simulink model "ThreePhaseVectorControl"  (R2020a)
settings: Solver=ode15s  StartTime=0.0  StopTime=2.5  MaxStep=1e-6  RelTol=1e-6
model workspace (MAT data in the model file):
  frequency = 1
values from neighbouring files (symbols this model uses):
  Buffer = 500    [PLLFYP.m]
  Ki_PLL = 0.005    [PLLFYP.m]
  Kp_PLL = 0.05    [PLLFYP.m]
  Kp_VSC = 500    [PLLFYP.m]
  Lf = 0.005    [PLLFYP.m]
  Lg = XR*Rg/(100*pi)    [PLLFYP.m]
  MPM_Ts = 1/5000    (= 0.0002)    [PLLFYP.m]
  Rf = 0.1    [PLLFYP.m]
  Rg = sqrt((1/(1+XR^2))*((500^2)/(Pn*SCR))^2)    [PLLFYP.m]
  Vdc = 2000    [PLLFYP.m]
  wL = 2*pi*50*Lf    (= 1.57079632679)    [PLLFYP.m]
  wn = 3000    [PLLFYP.m]
  zeta = 0.707    [PLLFYP.m]
undefined symbols (not defined in the file or in its folder): Ki_PQ, Kp_PQ, mpm_wc, plecs, Q, Q_KF, R, wb, wc, wc1, wc2
libraries: powerlib_meascontrol x57, powerlib x25, simulink x4, eeStairGenerator x4, powerlib_extras x2, cstblocks x2
(part 2 of 4)

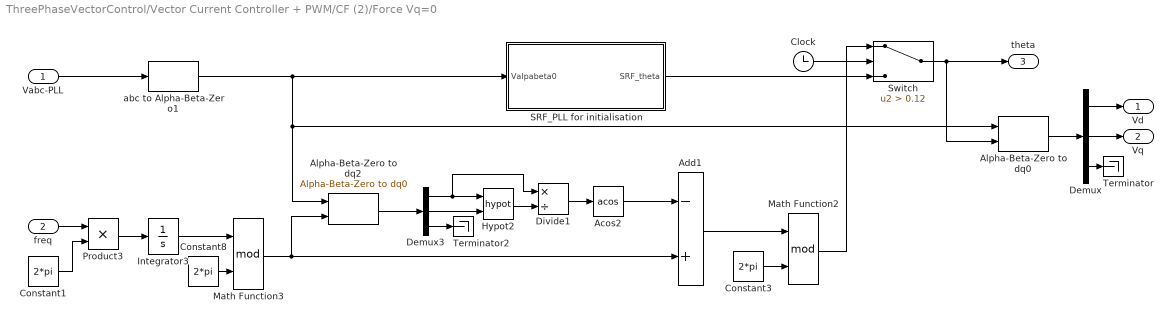
== system ThreePhaseVectorControl/Vector Current Controller + PWM/CF (2)/Force Vq=0 ==
  Vabc-PLL : Inport
  freq : Inport  Port=2
  Acos2 : Trigonometry  Operator=acos
  Add1 : Sum  Inputs=-+
  Alpha-Beta-Zero to dq0 : powerlib_meascontrol/Transformations/Alpha-Beta-Zero to dq0  Alignment=Aligned with phase A axis
  Alpha-Beta-Zero to dq2 : powerlib_meascontrol/Transformations/Alpha-Beta-Zero to dq0  Alignment=Aligned with phase A axis
  Clock : Clock
  Constant1 : Constant  Value=2*pi
  Constant3 : Constant  Value=2*pi
  Constant8 : Constant  Value=2*pi
  Demux : Demux  Outputs=3
  Demux3 : Demux  Outputs=3
  Divide1 : Product  Inputs=*/
  Hypot2 : Math  Operator=hypot  SaturateOnIntegerOverflow=on
  Integrator3 : Integrator  UpperSaturationLimit=2*pi  LowerSaturationLimit=0  IgnoreLimit=on
  Math Function2 : Math  Operator=mod  SignedPower=on  SaturateOnIntegerOverflow=on
  Math Function3 : Math  Operator=mod  SignedPower=on  SaturateOnIntegerOverflow=on
  Product3 : Product  RndMeth=Zero
  SRF_PLL for initialisation : Subsystem
  Switch : Switch  Criteria=u2 > Threshold  Threshold=0.12
  Terminator : Terminator
  Terminator2 : Terminator
  abc to Alpha-Beta-Zero1 : powerlib_meascontrol/Transformations/abc to Alpha-Beta-Zero
  Vd : Outport
  Vq : Outport  Port=2
  theta : Outport  Port=3  VectorParamsAs1DForOutWhenUnconnected=off
  wires:
  Add1/1 -> Math Function2/1
  Alpha-Beta-Zero to dq2/1 -> Demux3/1
  Demux3/3 -> Terminator2/1
  Constant3/1 -> Math Function2/2
  Math Function2/1 -> Switch/1
  Clock/1 -> Switch/2
  SRF_PLL for initialisation/1(SRF_theta) -> Switch/3
  Switch/1 -> theta/1, Alpha-Beta-Zero to dq0/2
  Divide1/1 -> Acos2/1
  Hypot2/1 -> Divide1/2
  Acos2/1 -> Add1/1
  Demux3/1 -> Hypot2/1, Divide1/1
  Demux3/2 -> Hypot2/2
  Vabc-PLL/1 -> abc to Alpha-Beta-Zero1/1
  Integrator3/1 -> Math Function3/1
  Constant1/1 -> Product3/2
  Product3/1 -> Integrator3/1
  Constant8/1 -> Math Function3/2
  freq/1 -> Product3/1
  Math Function3/1 -> Alpha-Beta-Zero to dq2/2, Add1/2
  abc to Alpha-Beta-Zero1/1 -> SRF_PLL for initialisation/1(Valpabeta0), Alpha-Beta-Zero to dq0/1, Alpha-Beta-Zero to dq2/1
  Alpha-Beta-Zero to dq0/1 -> Demux/1
  Demux/3 -> Terminator/1
  Demux/2 -> Vq/1
  Demux/1 -> Vd/1

== system ThreePhaseVectorControl/Vector Current Controller + PWM/CF (2)/MPM ==
  va : Inport
  Buffer : Buffer  N=Buffer  V=Overlap  ic=zeros(Buffer,1)  OutputFrames=off
  Clock3 : Clock
      settings: Decimation=100
  Constant : Constant  Value=Buffer/2
  Constant1 : Constant  Value=50
  Constant2 : Constant  Value=MPM_Ts
  Constant4 : Constant  Value=50
  MPM method : MATLAB Function  TreatAsAtomicUnit=on
  Scope2 : Scope
  Switch3 : Switch  Criteria=u2 > Threshold  Threshold=0.1
  Zero-Order Hold : ZeroOrderHold  SampleTime=MPM_Ts
  MPM freq : Outport
  wires:
  Constant/1 -> MPM method/2(L)
  Zero-Order Hold/1 -> Scope2/1, Buffer/1
  Constant1/1 -> MPM method/4(freq_guess)
  Buffer/1 -> MPM method/1(x)
  Clock3/1 -> Switch3/2
  Constant4/1 -> Switch3/3
  Constant2/1 -> MPM method/3(timestep)
  MPM method/1(outputfreq) -> Switch3/1
  va/1 -> Zero-Order Hold/1
  Switch3/1 -> MPM freq/1

== system ThreePhaseVectorControl/Vector Current Controller + PWM/CF (2)/SRF PLL ==
  Vabc : Inport
  1/(2*pi) : Step  Time=0  After=1/(2*pi)  SampleTime=0
  Add : Sum  Inputs=+-
  Add1 : Sum
  Constant : Constant  Value=2*pi
  Demux : Demux  Outputs=3
  Gain : Gain  Gain=Kp_PLL
  Integrator : Integrator  UpperSaturationLimit=2*pi  LowerSaturationLimit=0  IgnoreLimit=on
  Math Function : Math  Operator=mod  SignedPower=on  SaturateOnIntegerOverflow=on
  PI Controller : TransferFcn  Numerator=[1 Ki_PLL]  Denominator=[1 0]
  Product : Product  RndMeth=Zero
  Terminator : Terminator
  Terminator1 : Terminator
  abc to dq0 : powerlib_meascontrol/Transformations/abc to dq0  Alignment=Aligned with phase A axis
  q reference : Step  Time=0  After=0  SampleTime=0
  w0 : Step  Time=0  After=2*pi*50  SampleTime=0
  frequency : Outport
  delta_w0 : Outport  Port=2
  wires:
  Vabc/1 -> abc to dq0/1
  Integrator/1 -> Math Function/1
  Gain/1 -> PI Controller/1
  Add1/1 -> Product/2, Integrator/1
  Demux/2 -> Add/1
  w0/1 -> Add1/2
  q reference/1 -> Add/2
  1/(2*pi)/1 -> Product/1
  Product/1 -> frequency/1
  PI Controller/1 -> Add1/1, delta_w0/1
  Constant/1 -> Math Function/2
  Demux/3 -> Terminator/1
  Add/1 -> Gain/1
  abc to dq0/1 -> Demux/1
  Math Function/1 -> abc to dq0/2
  Demux/1 -> Terminator1/1

== system ThreePhaseVectorControl/Vector Current Controller + PWM/CF 2/MPM ==
  va : Inport
  Buffer : Buffer  N=500  V=499  ic=zeros(500,1)  OutputFrames=off
  Clock3 : Clock
      settings: Decimation=100
  Constant : Constant  Value=250
  Constant1 : Constant  Value=50
  Constant2 : Constant  Value=MPM_Ts
  Constant4 : Constant  Value=50
  MPM method : MATLAB Function  TreatAsAtomicUnit=on
  Scope2 : Scope
  Switch3 : Switch  Criteria=u2 > Threshold  Threshold=0.12
  Zero-Order Hold : ZeroOrderHold  SampleTime=MPM_Ts
  MPM freq : Outport
  wires:
  Constant/1 -> MPM method/2(L)
  Zero-Order Hold/1 -> Scope2/1, Buffer/1
  Constant1/1 -> MPM method/4(freq_guess)
  Buffer/1 -> MPM method/1(x)
  Clock3/1 -> Switch3/2
  Constant4/1 -> Switch3/3
  Constant2/1 -> MPM method/3(timestep)
  MPM method/1(outputfreq) -> Switch3/1
  va/1 -> Zero-Order Hold/1
  Switch3/1 -> MPM freq/1

== system ThreePhaseVectorControl/Vector Current Controller + PWM/CF 2/MPM (forcing Vq=0) ==
  Vabc-PLL : Inport
  MPM theta : Inport  Port=2
  Acos2 : Trigonometry  Operator=acos
  Add1 : Sum  Inputs=-+
  Alpha-Beta-Zero to dq2 : powerlib_meascontrol/Transformations/Alpha-Beta-Zero to dq0  Alignment=Aligned with phase A axis
  Clock : Clock
  Constant3 : Constant  Value=2*pi
  Demux3 : Demux  Outputs=3
  Divide1 : Product  Inputs=*/
  Hypot2 : Math  Operator=hypot  SaturateOnIntegerOverflow=on
  Math Function2 : Math  Operator=mod  SignedPower=on  SaturateOnIntegerOverflow=on
  SRF-PLL for initialization : Subsystem
  Switch : Switch  Criteria=u2 > Threshold  Threshold=0.12
  Terminator2 : Terminator
  abc to Alpha-Beta-Zero1 : powerlib_meascontrol/Transformations/abc to Alpha-Beta-Zero
  MPM_theta : Outport  VectorParamsAs1DForOutWhenUnconnected=off
  wires:
  Add1/1 -> Math Function2/1
  Alpha-Beta-Zero to dq2/1 -> Demux3/1
  Demux3/3 -> Terminator2/1
  Constant3/1 -> Math Function2/2
  Math Function2/1 -> Switch/1
  Clock/1 -> Switch/2
  SRF-PLL for initialization/1(SRF_theta) -> Switch/3
  abc to Alpha-Beta-Zero1/1 -> Alpha-Beta-Zero to dq2/1, SRF-PLL for initialization/1(VaB0)
  Switch/1 -> MPM_theta/1
  MPM theta/1 -> Alpha-Beta-Zero to dq2/2, Add1/2
  Divide1/1 -> Acos2/1
  Hypot2/1 -> Divide1/2
  Acos2/1 -> Add1/1
  Demux3/1 -> Hypot2/1, Divide1/1
  Demux3/2 -> Hypot2/2
  Vabc-PLL/1 -> abc to Alpha-Beta-Zero1/1

== system ThreePhaseVectorControl/Vector Current Controller + PWM/CF 2/SRF PLL ==
  abc : Inport
  wt : Inport  Port=2
  1/(2*pi) : Step  Time=0  After=1/(2*pi)  SampleTime=0
  Add : Sum  Inputs=+-
  Add1 : Sum
  Constant : Constant  Value=2*pi
  Demux : Demux  Outputs=3
  Gain : Gain  Gain=Kp_PLL
  Integrator : Integrator  UpperSaturationLimit=2*pi  LowerSaturationLimit=0  IgnoreLimit=on
  Math Function : Math  Operator=mod  SignedPower=on  SaturateOnIntegerOverflow=on
  PI Controller : TransferFcn  Numerator=[1 Ki_PLL]  Denominator=[1 0]
  Product : Product  RndMeth=Zero
  Terminator : Terminator
  abc to dq0 : powerlib_meascontrol/Transformations/abc to dq0  Alignment=Aligned with phase A axis
  q reference : Step  Time=0  After=0  SampleTime=0
  w0 : Step  Time=0  After=2*pi*50  SampleTime=0
  Vd : Outport  VectorParamsAs1DForOutWhenUnconnected=off
  Vq : Outport  Port=2  VectorParamsAs1DForOutWhenUnconnected=off
  delta_w0 : Outport  Port=3
  frequency : Outport  Port=4
  theta : Outport  Port=5
  wires:
  abc/1 -> abc to dq0/1
  Gain/1 -> PI Controller/1
  Add1/1 -> Integrator/1, Product/2
  Demux/2 -> Vq/1, Add/1
  w0/1 -> Add1/2
  Demux/1 -> Vd/1
  q reference/1 -> Add/2
  1/(2*pi)/1 -> Product/1
  Product/1 -> frequency/1
  PI Controller/1 -> Add1/1, delta_w0/1
  Demux/3 -> Terminator/1
  Add/1 -> Gain/1
  abc to dq0/1 -> Demux/1
  wt/1 -> abc to dq0/2
  Constant/1 -> Math Function/2
  Integrator/1 -> Math Function/1
  Math Function/1 -> theta/1

== system ThreePhaseVectorControl/Vector Current Controller + PWM/FFT_PLL/MPM (forcing Vq=0) ==
  Vabc-PLL : Inport
  FFT theta : Inport  Port=2
  Acos2 : Trigonometry  Operator=acos
  Add1 : Sum  Inputs=-+
  Alpha-Beta-Zero to dq2 : powerlib_meascontrol/Transformations/Alpha-Beta-Zero to dq0  Alignment=Aligned with phase A axis
  Alpha-Beta-Zero to dq3 : powerlib_meascontrol/Transformations/Alpha-Beta-Zero to dq0  Alignment=Aligned with phase A axis
  Clock : Clock
  Constant3 : Constant  Value=2*pi
  Demux3 : Demux  Outputs=3
  Demux4 : Demux  Outputs=3
  Divide1 : Product  Inputs=*/
  Hypot2 : Math  Operator=hypot  SaturateOnIntegerOverflow=on
  Math Function2 : Math  Operator=mod  SignedPower=on  SaturateOnIntegerOverflow=on
  SRF-PLL for initialization : Subsystem
  Switch : Switch  Criteria=u2 > Threshold  Threshold=0.12
  Terminator2 : Terminator
  Terminator3 : Terminator
  abc to Alpha-Beta-Zero1 : powerlib_meascontrol/Transformations/abc to Alpha-Beta-Zero
  FFT_theta : Outport  VectorParamsAs1DForOutWhenUnconnected=off
  Vd FFT : Outport  Port=2  VectorParamsAs1DForOutWhenUnconnected=off
  Vq FFT : Outport  Port=3  VectorParamsAs1DForOutWhenUnconnected=off
  wires:
  Add1/1 -> Math Function2/1
  Alpha-Beta-Zero to dq2/1 -> Demux3/1
  Demux3/3 -> Terminator2/1
  Constant3/1 -> Math Function2/2
  Math Function2/1 -> Switch/1, Alpha-Beta-Zero to dq3/2
  Demux4/3 -> Terminator3/1
  Alpha-Beta-Zero to dq3/1 -> Demux4/1
  Clock/1 -> Switch/2
  SRF-PLL for initialization/1(SRF_theta) -> Switch/3
  abc to Alpha-Beta-Zero1/1 -> Alpha-Beta-Zero to dq3/1, Alpha-Beta-Zero to dq2/1, SRF-PLL for initialization/1(VaB0)
  Switch/1 -> FFT_theta/1
  FFT theta/1 -> Alpha-Beta-Zero to dq2/2, Add1/2
  Divide1/1 -> Acos2/1
  Hypot2/1 -> Divide1/2
  Acos2/1 -> Add1/1
  Demux3/1 -> Hypot2/1, Divide1/1
  Demux3/2 -> Hypot2/2
  Vabc-PLL/1 -> abc to Alpha-Beta-Zero1/1
  Demux4/1 -> Vd FFT/1
  Demux4/2 -> Vq FFT/1

== system ThreePhaseVectorControl/Vector Current Controller + PWM/KF_PLL/KF//GAM ==
  Vabc : Inport
  " " : Constant  Value=R
  "  " : Constant  Value=Q_KF
  Clock3 : Clock
      settings: Decimation=100
  Constant1 : Constant  Value=2*pi
  Constant2 : Constant  Value=1/(2*pi)
  Constant4 : Constant  Value=2*pi*50
  Integrator1 : Integrator  UpperSaturationLimit=2*pi  LowerSaturationLimit=0  IgnoreLimit=on
  KF/GAM : Product
  Kalman Filter : Subsystem
  Math Function1 : Math  Operator=mod  SignedPower=on  SaturateOnIntegerOverflow=on
  Pulse Generator : DiscretePulseGenerator  PulseType=Time based  Period=10e-6  PulseWidth=50
  Real Time Frequency Detection : Subsystem
  Scope : Scope  NumInputPorts=2
  Switch3 : Switch  Criteria=u2 > Threshold  Threshold=0.12
  abc-to-aphabetazero and Normalized : Subsystem
  KF_f : Outport
  KF theta : Outport  Port=2
  wires:
  "  "/1 -> Kalman Filter/3(Q)
  Pulse Generator/1 -> Kalman Filter/Trigger, Real Time Frequency Detection/Trigger, abc-to-aphabetazero and Normalized/Trigger
  Kalman Filter/1(Vak_S90) -> abc-to-aphabetazero and Normalized/1(Va S90)
  Kalman Filter/2(Vbk_S90) -> abc-to-aphabetazero and Normalized/2(Vb S90)
  " "/1 -> Kalman Filter/2(R)
  abc-to-aphabetazero and Normalized/1(r_bw) -> Real Time Frequency Detection/1(r1), Scope/2
  abc-to-aphabetazero and Normalized/2(r_aw) -> Real Time Frequency Detection/2(r2), Scope/1
  Constant2/1 -> KF/GAM/2
  Kalman Filter/3(Vck_S90) -> abc-to-aphabetazero and Normalized/3(Vc S90)
  Integrator1/1 -> Math Function1/1
  Constant1/1 -> Math Function1/2
  Math Function1/1 -> KF theta/1
  KF/GAM/1 -> KF_f/1
  Clock3/1 -> Switch3/2
  Constant4/1 -> Switch3/3
  Vabc/1 -> Kalman Filter/1(Vabc)
  Real Time Frequency Detection/1(w_k) -> Switch3/1
  Switch3/1 -> Integrator1/1, Kalman Filter/4(w_k), KF/GAM/1

== system ThreePhaseVectorControl/Vector Current Controller + PWM/KF_PLL/Kalman Filter-based PLL ==
  note: $f (Hz)$
  vg_a : Inport
  vg_b : Inport  Port=2
  vg_c : Inport  Port=3
  " " : Constant  Value=500
  "  " : Constant  Value=0.05*eye(6)
  Constant : Constant  Value=0
  Constant2 : Constant  Value=1/(2*pi)
  Constant3 : Constant  Value=2*pi*50
  Kalman Filter : Subsystem
  Product7 : Product
  Pulse Generator : DiscretePulseGenerator  PulseType=Time based  Period=10e-6  PulseWidth=50
  Real Time Frequency Detection : Subsystem
  Scope : Scope  NumInputPorts=2
  Scope1 : Scope
  Scope5 : Scope
  abc-to-aphabetazero and Normalized : Subsystem
  powergui : powerlib/powergui  Priority=1  SimulationMode=Discrete  SampleTime=10e-6  frequency=60  Iterations=50  frequencyindice=60  Pbase=100e6  ErrMax=1e-4  UnitsV=kV  UnitsW=MW  buscounter=0  FunctionMessages=off  echomessages=off  EnableUseOfTLC=off  CurrentSourceSwitches=off  DisableSnubberDevices=off  DisableRonSwitches=off  DisableVfSwitches=off  DisplayEquations=off  AutomaticDiscreteSolvers=off  SolverType=Tustin/Backward Euler (TBE)  Interpol=off  ExternalGateDelay=off  methode=off  Ts=100  x0status=blocks  SPID=on  SwTol=0  HookPort=off  NonlinearTolerance=1e-4  nMaxIteration=100  ContinueOnMaxIteration=off  RestoreLinks=warning  ResistiveCurrentMeasurement=off  Frange=[0:2:500]  Ylog=off  Xlog=on  ShowGrid=off  save=off  variable=ZData  structure=0  ZoomFFT=off  StartTime=0.0  cycles=1  DisplayStyle=1  fundamental=60  FreqAxis=off  MaxFrequency=1000  frequencyindicesteady=1  RmsSteady=1  display=off
  wires:
  Constant2/1 -> Product7/2
  Product7/1 -> Scope5/1
  " "/1 -> Kalman Filter/4(R)
  "  "/1 -> Kalman Filter/5(Q)
  Constant/1 -> Kalman Filter/6(w_fk)
  Kalman Filter/1(Vak_S90) -> abc-to-aphabetazero and Normalized/1(Va S90)
  Kalman Filter/2(Vbk_S90) -> abc-to-aphabetazero and Normalized/2(Vb S90)
  Kalman Filter/3(Vck_S90) -> abc-to-aphabetazero and Normalized/3(Vc S90)
  vg_a/1 -> Kalman Filter/1(Va)
  vg_b/1 -> Kalman Filter/2(Vb)
  vg_c/1 -> Kalman Filter/3(Vc)
  Pulse Generator/1 -> Real Time Frequency Detection/Trigger, abc-to-aphabetazero and Normalized/Trigger, Kalman Filter/Trigger
  abc-to-aphabetazero and Normalized/2(r_aw) -> Real Time Frequency Detection/2(r2), Scope/1
  abc-to-aphabetazero and Normalized/1(r_bw) -> Real Time Frequency Detection/1(r1), Scope/2
  Real Time Frequency Detection/1(w_k) -> Scope1/1, Product7/1
  Constant3/1 -> Kalman Filter/7(w_k)

== system ThreePhaseVectorControl/Vector Current Controller + PWM/KF_PLL/MPM (forcing Vq=0) ==
  Vabc-PLL : Inport
  KF theta : Inport  Port=2
  Acos2 : Trigonometry  Operator=acos
  Add1 : Sum  Inputs=-+
  Alpha-Beta-Zero to dq2 : powerlib_meascontrol/Transformations/Alpha-Beta-Zero to dq0  Alignment=Aligned with phase A axis
  Alpha-Beta-Zero to dq3 : powerlib_meascontrol/Transformations/Alpha-Beta-Zero to dq0  Alignment=Aligned with phase A axis
  Clock : Clock
  Constant3 : Constant  Value=2*pi
  Demux3 : Demux  Outputs=3
  Demux4 : Demux  Outputs=3
  Divide1 : Product  Inputs=*/
  Hypot2 : Math  Operator=hypot  SaturateOnIntegerOverflow=on
  Math Function2 : Math  Operator=mod  SignedPower=on  SaturateOnIntegerOverflow=on
  SRF-PLL for initialization : Subsystem
  Switch : Switch  Criteria=u2 > Threshold  Threshold=0.12
  Terminator2 : Terminator
  Terminator3 : Terminator
  abc to Alpha-Beta-Zero1 : powerlib_meascontrol/Transformations/abc to Alpha-Beta-Zero
  KF_theta : Outport  VectorParamsAs1DForOutWhenUnconnected=off
  Vd KF : Outport  Port=2  VectorParamsAs1DForOutWhenUnconnected=off
  Vq KF : Outport  Port=3  VectorParamsAs1DForOutWhenUnconnected=off
  wires:
  Add1/1 -> Math Function2/1
  Alpha-Beta-Zero to dq2/1 -> Demux3/1
  Demux3/3 -> Terminator2/1
  Constant3/1 -> Math Function2/2
  Math Function2/1 -> Switch/1, Alpha-Beta-Zero to dq3/2
  Demux4/3 -> Terminator3/1
  Alpha-Beta-Zero to dq3/1 -> Demux4/1
  Clock/1 -> Switch/2
  SRF-PLL for initialization/1(SRF_theta) -> Switch/3
  abc to Alpha-Beta-Zero1/1 -> Alpha-Beta-Zero to dq3/1, Alpha-Beta-Zero to dq2/1, SRF-PLL for initialization/1(VaB0)
  Switch/1 -> KF_theta/1
  KF theta/1 -> Add1/2, Alpha-Beta-Zero to dq2/2
  Divide1/1 -> Acos2/1
  Hypot2/1 -> Divide1/2
  Acos2/1 -> Add1/1
  Demux3/1 -> Hypot2/1, Divide1/1
  Demux3/2 -> Hypot2/2
  Demux4/2 -> Vq KF/1
  Demux4/1 -> Vd KF/1
  Vabc-PLL/1 -> abc to Alpha-Beta-Zero1/1

== system ThreePhaseVectorControl/Vector Current Controller + PWM/MPM/MPM ==
  va : Inport
  2*pi3 : Step  Time=0  After=2*pi  SampleTime=0
  Buffer : Buffer  N=Buffer  V=Overlap  ic=zeros(Buffer,1)  OutputFrames=off
  Clock3 : Clock
      settings: Decimation=100
  Constant : Constant  Value=Buffer/2
  Constant1 : Constant  Value=50
  Constant2 : Constant  Value=MPM_Ts
  Constant4 : Constant  Value=50
  Constant8 : Constant  Value=2*pi
  Integrator3 : Integrator  UpperSaturationLimit=2*pi  LowerSaturationLimit=0  IgnoreLimit=on
  MPM method : MATLAB Function  TreatAsAtomicUnit=on
  Math Function3 : Math  Operator=mod  SignedPower=on  SaturateOnIntegerOverflow=on
  Product3 : Product  RndMeth=Zero
  Scope2 : Scope
  Switch3 : Switch  Criteria=u2 > Threshold  Threshold=0.12
  Zero-Order Hold : ZeroOrderHold  SampleTime=MPM_Ts
  freq : Outport
  MPM theta : Outport  Port=2
  wires:
  Constant/1 -> MPM method/2(L)
  Zero-Order Hold/1 -> Scope2/1, Buffer/1
  Constant1/1 -> MPM method/4(freq_guess)
  Buffer/1 -> MPM method/1(x)
  Clock3/1 -> Switch3/2
  Constant4/1 -> Switch3/3
  Constant2/1 -> MPM method/3(timestep)
  Constant8/1 -> Math Function3/2
  2*pi3/1 -> Product3/2
  Switch3/1 -> freq/1, Product3/1
  MPM method/1(outputfreq) -> Switch3/1
  va/1 -> Zero-Order Hold/1
  Product3/1 -> Integrator3/1
  Integrator3/1 -> Math Function3/1
  Math Function3/1 -> MPM theta/1

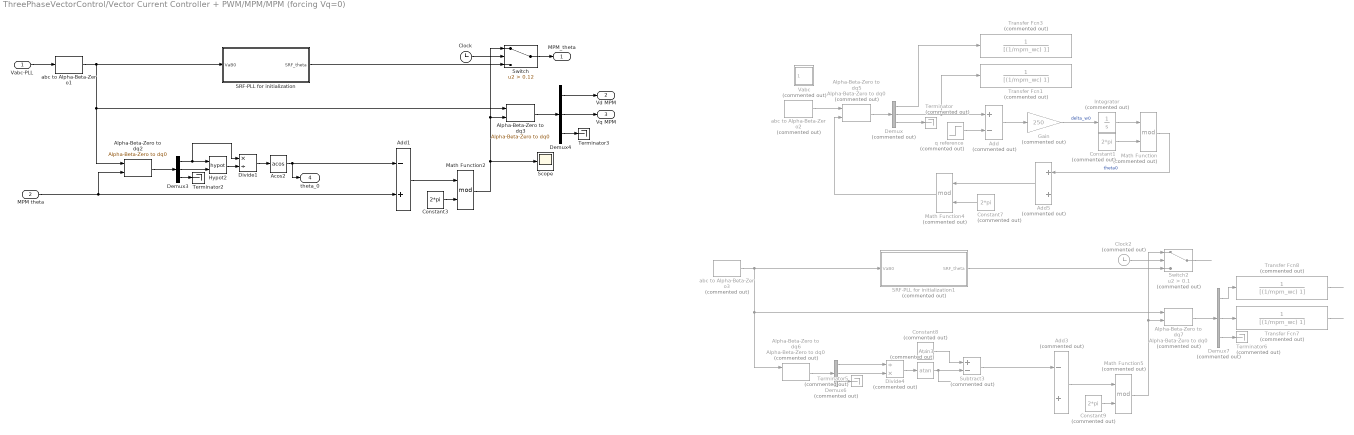
== system ThreePhaseVectorControl/Vector Current Controller + PWM/MPM/MPM (forcing Vq=0) ==
  Vabc-PLL : Inport
  MPM theta : Inport  Port=2
  Acos2 : Trigonometry  Operator=acos
  Add : Sum  Commented=on  Inputs=+-
  Add1 : Sum  Inputs=-+
  Add3 : Sum  Commented=on  Inputs=-+
  Add5 : Sum  Commented=on
  Alpha-Beta-Zero to dq2 : powerlib_meascontrol/Transformations/Alpha-Beta-Zero to dq0  Alignment=Aligned with phase A axis
  Alpha-Beta-Zero to dq3 : powerlib_meascontrol/Transformations/Alpha-Beta-Zero to dq0  Alignment=Aligned with phase A axis
  Alpha-Beta-Zero to dq5 : powerlib_meascontrol/Transformations/Alpha-Beta-Zero to dq0  Commented=on  Alignment=Aligned with phase A axis
  Alpha-Beta-Zero to dq6 : powerlib_meascontrol/Transformations/Alpha-Beta-Zero to dq0  Commented=on  Alignment=Aligned with phase A axis
  Alpha-Beta-Zero to dq7 : powerlib_meascontrol/Transformations/Alpha-Beta-Zero to dq0  Commented=on  Alignment=Aligned with phase A axis
  Atan3 : Trigonometry  Commented=on  Operator=atan
  Clock : Clock
  Clock2 : Clock  Commented=on
  Constant1 : Constant  Commented=on  Value=2*pi
  Constant3 : Constant  Value=2*pi
  Constant7 : Constant  Commented=on  Value=2*pi
  Constant8 : Constant  Commented=on  Value=pi
  Constant9 : Constant  Commented=on  Value=2*pi
  Demux : Demux  Commented=on  Outputs=3
  Demux3 : Demux  Outputs=3
  Demux4 : Demux  Outputs=3
  Demux6 : Demux  Commented=on  Outputs=3
  Demux7 : Demux  Commented=on  Outputs=3
  Divide1 : Product  Inputs=*/
  Divide4 : Product  Commented=on  Inputs=/*
  Gain : Gain  Commented=on  Gain=250
  Hypot2 : Math  Operator=hypot  SaturateOnIntegerOverflow=on
  Integrator : Integrator  Commented=on  UpperSaturationLimit=2*pi  LowerSaturationLimit=0  IgnoreLimit=on
  Math Function : Math  Commented=on  Operator=mod  SignedPower=on  SaturateOnIntegerOverflow=on
  Math Function2 : Math  Operator=mod  SignedPower=on  SaturateOnIntegerOverflow=on
  Math Function4 : Math  Commented=on  Operator=mod  SignedPower=on  SaturateOnIntegerOverflow=on
  Math Function5 : Math  Commented=on  Operator=mod  SignedPower=on  SaturateOnIntegerOverflow=on
  SRF-PLL for initialization : Subsystem
  SRF-PLL for initialization1 : Subsystem  Commented=on
  Scope : Scope
  Subtract3 : Sum  Commented=on  Inputs=+-
  Switch : Switch  Criteria=u2 > Threshold  Threshold=0.12
  Switch2 : Switch  Commented=on  Criteria=u2 > Threshold  Threshold=0.1
  Terminator : Terminator  Commented=on
  Terminator2 : Terminator
  Terminator3 : Terminator
  Terminator5 : Terminator  Commented=on
  Terminator6 : Terminator  Commented=on
  Transfer Fcn{1,3,7..8} (4 alike) : TransferFcn  Commented=on  Denominator=[(1/mpm_wc) 1]
  Vabc : Subsystem  Commented=on  LoadFcn=plecs('sl', 300);  InitFcn=plecs('sl', 314);  StartFcn=plecs('sl', 308);  StopFcn=plecs('sl', 309);  mask{Settings=<binary blob, 236 chars, not shown>}
      mask init:
      | plecs('sl', 315);
      settings: CopyFcn=plecs('sl', 303);  DeleteFcn=plecs('sl', 305);  UndoDeleteFcn=plecs('sl', 306);  PreSaveFcn=plecs('sl', 311);  NameChangeFcn=plecs('sl', 310);  DestroyFcn=plecs('sl', 307);  OpenFcn=plecs('sl', 302);  ErrorFcn=plerrorfcn
      mask Display: plot([0.1 0.9 0.9 0.1 0.1], [0.9 0.9 0.5 0.5 0.9])
  abc to Alpha-Beta-Zero1 : powerlib_meascontrol/Transformations/abc to Alpha-Beta-Zero
  abc to Alpha-Beta-Zero2 : powerlib_meascontrol/Transformations/abc to Alpha-Beta-Zero  Commented=on
  abc to Alpha-Beta-Zero3 : powerlib_meascontrol/Transformations/abc to Alpha-Beta-Zero  Commented=on
  q reference : Step  Commented=on  Time=0  After=0  SampleTime=0
  MPM_theta : Outport  VectorParamsAs1DForOutWhenUnconnected=off
  Vd MPM : Outport  Port=2  VectorParamsAs1DForOutWhenUnconnected=off
  Vq MPM : Outport  Port=3  VectorParamsAs1DForOutWhenUnconnected=off
  theta_0 : Outport  Port=4
  wires:
  Add1/1 -> Math Function2/1
  Alpha-Beta-Zero to dq2/1 -> Demux3/1
  Demux3/3 -> Terminator2/1
  Constant3/1 -> Math Function2/2
  Demux/3 -> Terminator/1
  Add/1 -> Gain/1
  Demux/2 -> Add/1, Transfer Fcn1/1
  Constant1/1 -> Math Function/2
  q reference/1 -> Add/2
  Gain/1 -> Integrator/1  "delta_w0"
  Math Function2/1 -> Scope/1, Switch/1, Alpha-Beta-Zero to dq3/2
  Demux4/3 -> Terminator3/1
  Alpha-Beta-Zero to dq3/1 -> Demux4/1
  Clock/1 -> Switch/2
  SRF-PLL for initialization/1(SRF_theta) -> Switch/3
  abc to Alpha-Beta-Zero1/1 -> Alpha-Beta-Zero to dq3/1, Alpha-Beta-Zero to dq2/1, SRF-PLL for initialization/1(VaB0)
  Integrator/1 -> Math Function/1
  Math Function/1 -> Add5/1  "theta0"
  Constant7/1 -> Math Function4/2
  Add5/1 -> Math Function4/1
  Demux/1 -> Transfer Fcn3/1
  Alpha-Beta-Zero to dq5/1 -> Demux/1
  Math Function4/1 -> Alpha-Beta-Zero to dq5/2
  abc to Alpha-Beta-Zero2/1 -> Alpha-Beta-Zero to dq5/1
  Switch/1 -> MPM_theta/1
  MPM theta/1 -> Alpha-Beta-Zero to dq2/2, Add1/2
  Constant9/1 -> Math Function5/2
  Alpha-Beta-Zero to dq6/1 -> Demux6/1
  Transfer Fcn8/1 -> ?
  Demux6/3 -> Terminator5/1
  Demux6/1 -> Divide4/1
  Switch2/1 -> ?
  ? -> abc to Alpha-Beta-Zero3/1
  ? -> Alpha-Beta-Zero to dq6/2, Add3/2
  Demux7/1 -> Transfer Fcn8/1
  Transfer Fcn7/1 -> ?
  Constant8/1 -> Subtract3/1
  Atan3/1 -> Subtract3/2
  Math Function5/1 -> Switch2/1, Alpha-Beta-Zero to dq7/2
  Add3/1 -> Math Function5/1
  Demux6/2 -> Divide4/2
  Clock2/1 -> Switch2/2
  Divide4/1 -> Atan3/1
  SRF-PLL for initialization1/1(SRF_theta) -> Switch2/3
  Demux7/2 -> Transfer Fcn7/1
  Subtract3/1 -> Add3/1
  abc to Alpha-Beta-Zero3/1 -> Alpha-Beta-Zero to dq7/1, Alpha-Beta-Zero to dq6/1, SRF-PLL for initialization1/1(VaB0)
  Alpha-Beta-Zero to dq7/1 -> Demux7/1
  Demux7/3 -> Terminator6/1
  Divide1/1 -> Acos2/1
  Hypot2/1 -> Divide1/2
  Acos2/1 -> Add1/1, theta_0/1
  Demux3/1 -> Hypot2/1, Divide1/1
  Demux3/2 -> Hypot2/2
  Vabc-PLL/1 -> abc to Alpha-Beta-Zero1/1
  Demux4/1 -> Vd MPM/1
  Demux4/2 -> Vq MPM/1

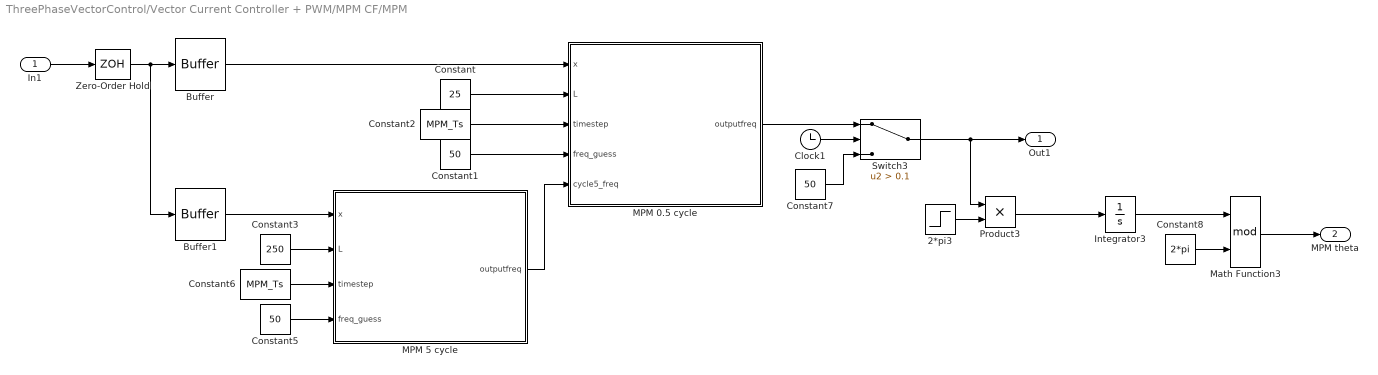
== system ThreePhaseVectorControl/Vector Current Controller + PWM/MPM CF/MPM ==
  In1 : Inport
  2*pi3 : Step  Time=0  After=2*pi  SampleTime=0
  Buffer : Buffer  N=50  V=49  ic=zeros(50,1)  OutputFrames=off
  Buffer1 : Buffer  N=500  V=499  ic=zeros(500,1)  OutputFrames=off
  Clock1 : Clock
      settings: Decimation=100
  Constant : Constant  Value=25
  Constant1 : Constant  Value=50
  Constant2 : Constant  Value=MPM_Ts
  Constant3 : Constant  Value=250
  Constant5 : Constant  Value=50
  Constant6 : Constant  Value=MPM_Ts
  Constant7 : Constant  Value=50
  Constant8 : Constant  Value=2*pi
  Integrator3 : Integrator  InitialCondition=0.000000001  UpperSaturationLimit=2*pi  LowerSaturationLimit=0  IgnoreLimit=on
  MPM 0.5 cycle : MATLAB Function  TreatAsAtomicUnit=on
  MPM 5 cycle : MATLAB Function  TreatAsAtomicUnit=on
  Math Function3 : Math  Operator=mod  SignedPower=on  SaturateOnIntegerOverflow=on
  Product3 : Product  RndMeth=Zero
  Switch3 : Switch  Criteria=u2 > Threshold  Threshold=0.1
  Zero-Order Hold : ZeroOrderHold  SampleTime=MPM_Ts
  Out1 : Outport
  MPM theta : Outport  Port=2
  wires:
  Math Function3/1 -> MPM theta/1
  Constant/1 -> MPM 0.5 cycle/2(L)
  Zero-Order Hold/1 -> Buffer1/1, Buffer/1
  Constant1/1 -> MPM 0.5 cycle/4(freq_guess)
  Buffer/1 -> MPM 0.5 cycle/1(x)
  Constant2/1 -> MPM 0.5 cycle/3(timestep)
  Constant8/1 -> Math Function3/2
  2*pi3/1 -> Product3/2
  Switch3/1 -> Product3/1, Out1/1
  In1/1 -> Zero-Order Hold/1
  Integrator3/1 -> Math Function3/1
  Product3/1 -> Integrator3/1
  Buffer1/1 -> MPM 5 cycle/1(x)
  Constant3/1 -> MPM 5 cycle/2(L)
  Constant5/1 -> MPM 5 cycle/4(freq_guess)
  Constant6/1 -> MPM 5 cycle/3(timestep)
  Clock1/1 -> Switch3/2
  MPM 0.5 cycle/1(outputfreq) -> Switch3/1
  Constant7/1 -> Switch3/3
  MPM 5 cycle/1(outputfreq) -> MPM 0.5 cycle/5(cycle5_freq)

== system ThreePhaseVectorControl/Vector Current Controller + PWM/MPM CF/MPM (forcing Vq=0) ==
  Vabc-PLL : Inport
  MPM theta : Inport  Port=2
  Acos2 : Trigonometry  Operator=acos
  Add1 : Sum  Inputs=-+
  Alpha-Beta-Zero to dq2 : powerlib_meascontrol/Transformations/Alpha-Beta-Zero to dq0  Alignment=Aligned with phase A axis
  Alpha-Beta-Zero to dq3 : powerlib_meascontrol/Transformations/Alpha-Beta-Zero to dq0  Alignment=Aligned with phase A axis
  Clock : Clock
  Constant3 : Constant  Value=2*pi
  Demux3 : Demux  Outputs=3
  Demux4 : Demux  Outputs=3
  Divide1 : Product  Inputs=*/
  Hypot2 : Math  Operator=hypot  SaturateOnIntegerOverflow=on
  Math Function2 : Math  Operator=mod  SignedPower=on  SaturateOnIntegerOverflow=on
  SRF-PLL for initialization : Subsystem
  Switch : Switch  Criteria=u2 > Threshold  Threshold=0.1
  Terminator2 : Terminator
  Terminator3 : Terminator
  abc to Alpha-Beta-Zero1 : powerlib_meascontrol/Transformations/abc to Alpha-Beta-Zero
  MPM_theta : Outport  VectorParamsAs1DForOutWhenUnconnected=off
  Vd MPM : Outport  Port=2  VectorParamsAs1DForOutWhenUnconnected=off
  Vq MPM : Outport  Port=3  VectorParamsAs1DForOutWhenUnconnected=off
  wires:
  Add1/1 -> Math Function2/1
  Alpha-Beta-Zero to dq2/1 -> Demux3/1
  Demux3/3 -> Terminator2/1
  Constant3/1 -> Math Function2/2
  Math Function2/1 -> Switch/1, Alpha-Beta-Zero to dq3/2
  Demux4/3 -> Terminator3/1
  Alpha-Beta-Zero to dq3/1 -> Demux4/1
  Clock/1 -> Switch/2
  SRF-PLL for initialization/1(SRF_theta) -> Switch/3
  abc to Alpha-Beta-Zero1/1 -> Alpha-Beta-Zero to dq3/1, Alpha-Beta-Zero to dq2/1, SRF-PLL for initialization/1(VaB0)
  Switch/1 -> MPM_theta/1
  MPM theta/1 -> Alpha-Beta-Zero to dq2/2, Add1/2
  Divide1/1 -> Acos2/1
  Hypot2/1 -> Divide1/2
  Acos2/1 -> Add1/1
  Demux3/1 -> Hypot2/1, Divide1/1
  Demux3/2 -> Hypot2/2
  Vabc-PLL/1 -> abc to Alpha-Beta-Zero1/1
  Demux4/1 -> Vd MPM/1
  Demux4/2 -> Vq MPM/1

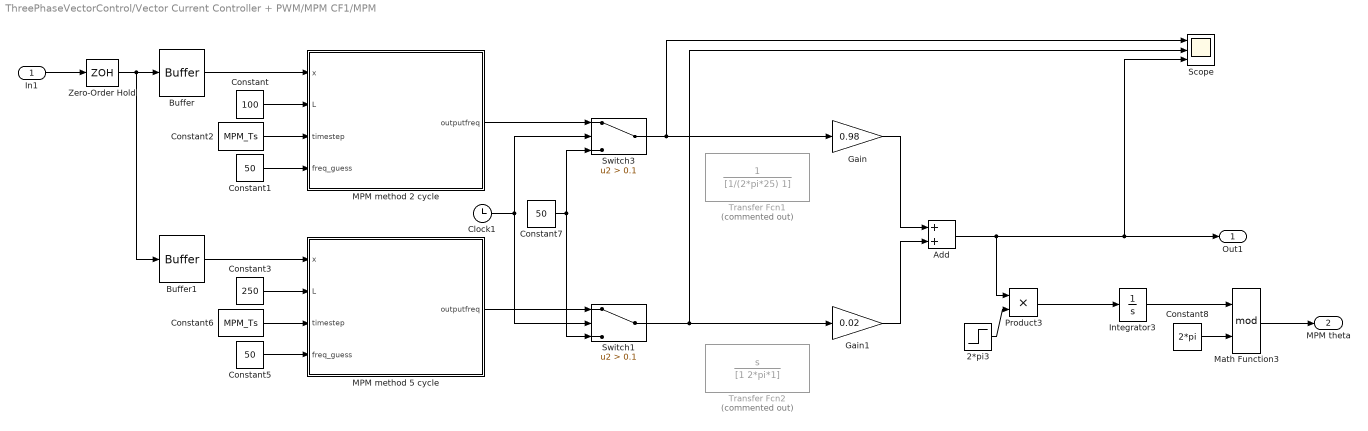
== system ThreePhaseVectorControl/Vector Current Controller + PWM/MPM CF1/MPM ==
  In1 : Inport
  2*pi3 : Step  Time=0  After=2*pi  SampleTime=0
  Add : Sum
  Buffer : Buffer  N=200  ic=zeros(200,1)  OutputFrames=off
  Buffer1 : Buffer  N=500  ic=zeros(500,1)  OutputFrames=off
  Clock1 : Clock
      settings: Decimation=100
  Constant : Constant  Value=100
  Constant1 : Constant  Value=50
  Constant2 : Constant  Value=MPM_Ts
  Constant3 : Constant  Value=250
  Constant5 : Constant  Value=50
  Constant6 : Constant  Value=MPM_Ts
  Constant7 : Constant  Value=50
  Constant8 : Constant  Value=2*pi
  Gain : Gain  Gain=0.98
  Gain1 : Gain  Gain=0.02
  Integrator3 : Integrator  InitialCondition=0.000000001  UpperSaturationLimit=2*pi  LowerSaturationLimit=0  IgnoreLimit=on
  MPM method 2 cycle : MATLAB Function  TreatAsAtomicUnit=on
  MPM method 5 cycle : MATLAB Function  TreatAsAtomicUnit=on
  Math Function3 : Math  Operator=mod  SignedPower=on  SaturateOnIntegerOverflow=on
  Product3 : Product  RndMeth=Zero
  Scope : Scope  NumInputPorts=3
  Switch1 : Switch  Criteria=u2 > Threshold  Threshold=0.1
  Switch3 : Switch  Criteria=u2 > Threshold  Threshold=0.1
  Transfer Fcn1 : TransferFcn  Commented=on  Denominator=[1/(2*pi*25) 1]
  Transfer Fcn2 : TransferFcn  Commented=on  Numerator=[1 0]  Denominator=[1 2*pi*1]
  Zero-Order Hold : ZeroOrderHold  SampleTime=MPM_Ts
  Out1 : Outport
  MPM theta : Outport  Port=2
  wires:
  Math Function3/1 -> MPM theta/1
  Constant/1 -> MPM method 2 cycle/2(L)
  Zero-Order Hold/1 -> Buffer1/1, Buffer/1
  Constant1/1 -> MPM method 2 cycle/4(freq_guess)
  Buffer/1 -> MPM method 2 cycle/1(x)
  Constant2/1 -> MPM method 2 cycle/3(timestep)
  Constant8/1 -> Math Function3/2
  2*pi3/1 -> Product3/2
  Add/1 -> Scope/3, Out1/1, Product3/1
  In1/1 -> Zero-Order Hold/1
  Integrator3/1 -> Math Function3/1
  Product3/1 -> Integrator3/1
  Buffer1/1 -> MPM method 5 cycle/1(x)
  Constant3/1 -> MPM method 5 cycle/2(L)
  Constant5/1 -> MPM method 5 cycle/4(freq_guess)
  Constant6/1 -> MPM method 5 cycle/3(timestep)
  Gain1/1 -> Add/2
  Gain/1 -> Add/1
  Clock1/1 -> Switch3/2, Switch1/2
  MPM method 2 cycle/1(outputfreq) -> Switch3/1
  Constant7/1 -> Switch3/3, Switch1/3
  MPM method 5 cycle/1(outputfreq) -> Switch1/1
  Switch1/1 -> Gain1/1, Scope/2
  Switch3/1 -> Gain/1, Scope/1

== system ThreePhaseVectorControl/Vector Current Controller + PWM/MPM CF1/MPM (forcing Vq=0) ==
  Vabc-PLL : Inport
  MPM theta : Inport  Port=2
  Acos2 : Trigonometry  Operator=acos
  Add1 : Sum  Inputs=-+
  Alpha-Beta-Zero to dq2 : powerlib_meascontrol/Transformations/Alpha-Beta-Zero to dq0  Alignment=Aligned with phase A axis
  Alpha-Beta-Zero to dq3 : powerlib_meascontrol/Transformations/Alpha-Beta-Zero to dq0  Alignment=Aligned with phase A axis
  Clock : Clock
  Constant3 : Constant  Value=2*pi
  Demux3 : Demux  Outputs=3
  Demux4 : Demux  Outputs=3
  Divide1 : Product  Inputs=*/
  Hypot2 : Math  Operator=hypot  SaturateOnIntegerOverflow=on
  Math Function2 : Math  Operator=mod  SignedPower=on  SaturateOnIntegerOverflow=on
  SRF-PLL for initialization : Subsystem
  Switch : Switch  Criteria=u2 > Threshold  Threshold=0.1
  Terminator2 : Terminator
  Terminator3 : Terminator
  abc to Alpha-Beta-Zero1 : powerlib_meascontrol/Transformations/abc to Alpha-Beta-Zero
  MPM_theta : Outport  VectorParamsAs1DForOutWhenUnconnected=off
  Vd MPM : Outport  Port=2  VectorParamsAs1DForOutWhenUnconnected=off
  Vq MPM : Outport  Port=3  VectorParamsAs1DForOutWhenUnconnected=off
  wires:
  Add1/1 -> Math Function2/1
  Alpha-Beta-Zero to dq2/1 -> Demux3/1
  Demux3/3 -> Terminator2/1
  Constant3/1 -> Math Function2/2
  Math Function2/1 -> Switch/1, Alpha-Beta-Zero to dq3/2
  Demux4/3 -> Terminator3/1
  Alpha-Beta-Zero to dq3/1 -> Demux4/1
  Clock/1 -> Switch/2
  SRF-PLL for initialization/1(SRF_theta) -> Switch/3
  abc to Alpha-Beta-Zero1/1 -> Alpha-Beta-Zero to dq3/1, Alpha-Beta-Zero to dq2/1, SRF-PLL for initialization/1(VaB0)
  Switch/1 -> MPM_theta/1
  MPM theta/1 -> Alpha-Beta-Zero to dq2/2, Add1/2
  Divide1/1 -> Acos2/1
  Hypot2/1 -> Divide1/2
  Acos2/1 -> Add1/1
  Demux3/1 -> Hypot2/1, Divide1/1
  Demux3/2 -> Hypot2/2
  Vabc-PLL/1 -> abc to Alpha-Beta-Zero1/1
  Demux4/1 -> Vd MPM/1
  Demux4/2 -> Vq MPM/1

== system ThreePhaseVectorControl/Vector Current Controller + PWM/MPM//SRF CF/MPM ==
  v_g : Inport
  Buffer1 : Buffer  N=500  ic=zeros(500,1)  OutputFrames=off
  Clock1 : Clock
      settings: Decimation=100
  Constant3 : Constant  Value=250
  Constant5 : Constant  Value=50
  Constant6 : Constant  Value=MPM_Ts
  Constant7 : Constant  Value=50
  MPM method 5 cycle : MATLAB Function  TreatAsAtomicUnit=on
  Switch1 : Switch  Criteria=u2 > Threshold  Threshold=0.1
  Zero-Order Hold : ZeroOrderHold  SampleTime=MPM_Ts
  MPM freq : Outport
  wires:
  Zero-Order Hold/1 -> Buffer1/1
  Buffer1/1 -> MPM method 5 cycle/1(x)
  Constant3/1 -> MPM method 5 cycle/2(L)
  Constant5/1 -> MPM method 5 cycle/4(freq_guess)
  Constant6/1 -> MPM method 5 cycle/3(timestep)
  Clock1/1 -> Switch1/2
  Constant7/1 -> Switch1/3
  MPM method 5 cycle/1(outputfreq) -> Switch1/1
  v_g/1 -> Zero-Order Hold/1
  Switch1/1 -> MPM freq/1  "MPM freq"

== system ThreePhaseVectorControl/Vector Current Controller + PWM/MPM//SRF CF/MPM (forcing Vq=0) ==
  Vabc-PLL : Inport
  CF theta : Inport  Port=2
  Acos2 : Trigonometry  Operator=acos
  Add1 : Sum  Inputs=-+
  Alpha-Beta-Zero to dq2 : powerlib_meascontrol/Transformations/Alpha-Beta-Zero to dq0  Alignment=Aligned with phase A axis
  Alpha-Beta-Zero to dq3 : powerlib_meascontrol/Transformations/Alpha-Beta-Zero to dq0  Alignment=Aligned with phase A axis
  Clock : Clock
  Constant3 : Constant  Value=2*pi
  Demux3 : Demux  Outputs=3
  Demux4 : Demux  Outputs=3
  Divide1 : Product  Inputs=*/
  Hypot2 : Math  Operator=hypot  SaturateOnIntegerOverflow=on
  Math Function2 : Math  Operator=mod  SignedPower=on  SaturateOnIntegerOverflow=on
  SRF-PLL for initialization : Subsystem
  Switch : Switch  Criteria=u2 > Threshold  Threshold=0.1
  Terminator2 : Terminator
  Terminator3 : Terminator
  abc to Alpha-Beta-Zero1 : powerlib_meascontrol/Transformations/abc to Alpha-Beta-Zero
  CF_theta : Outport  VectorParamsAs1DForOutWhenUnconnected=off
  Vd CF : Outport  Port=2  VectorParamsAs1DForOutWhenUnconnected=off
  Vq CF : Outport  Port=3  VectorParamsAs1DForOutWhenUnconnected=off
  wires:
  Add1/1 -> Math Function2/1
  Alpha-Beta-Zero to dq2/1 -> Demux3/1
  Demux3/3 -> Terminator2/1
  Constant3/1 -> Math Function2/2
  Math Function2/1 -> Switch/1, Alpha-Beta-Zero to dq3/2
  Demux4/3 -> Terminator3/1
  Alpha-Beta-Zero to dq3/1 -> Demux4/1
  Clock/1 -> Switch/2
  SRF-PLL for initialization/1(SRF_theta) -> Switch/3
  abc to Alpha-Beta-Zero1/1 -> Alpha-Beta-Zero to dq3/1, Alpha-Beta-Zero to dq2/1, SRF-PLL for initialization/1(VaB0)
  Switch/1 -> CF_theta/1
  CF theta/1 -> Alpha-Beta-Zero to dq2/2, Add1/2
  Divide1/1 -> Acos2/1
  Hypot2/1 -> Divide1/2
  Acos2/1 -> Add1/1
  Demux3/1 -> Hypot2/1, Divide1/1
  Demux3/2 -> Hypot2/2
  Vabc-PLL/1 -> abc to Alpha-Beta-Zero1/1
  Demux4/1 -> Vd CF/1
  Demux4/2 -> Vq CF/1

== system ThreePhaseVectorControl/Vector Current Controller + PWM/MPM//SRF CF/SRF_PLL ==
  Vabc-PLL : Inport
  1/(2*pi) : Step  Time=0  After=1/(2*pi)  SampleTime=0
  Add : Sum  Inputs=+-
  Add1 : Sum
  Alpha-Beta-Zero to dq0 : powerlib_meascontrol/Transformations/Alpha-Beta-Zero to dq0  Alignment=Aligned with phase A axis
  Constant : Constant  Value=2*pi
  Demux : Demux  Outputs=3
  Gain : Gain  Gain=Kp_PLL
  Integrator : Integrator  UpperSaturationLimit=2*pi  LowerSaturationLimit=0  IgnoreLimit=on
  Math Function : Math  Operator=mod  SignedPower=on  SaturateOnIntegerOverflow=on
  PI Controller : TransferFcn  Numerator=[1 Ki_PLL]  Denominator=[1 0]
  Product : Product  RndMeth=Zero
  Terminator : Terminator
  Terminator1 : Terminator
  Vabc : Subsystem  Commented=on  LoadFcn=plecs('sl', 300);  InitFcn=plecs('sl', 314);  StartFcn=plecs('sl', 308);  StopFcn=plecs('sl', 309);  mask{Settings=<binary blob, 236 chars, not shown>}
      mask init:
      | plecs('sl', 315);
      settings: CopyFcn=plecs('sl', 303);  DeleteFcn=plecs('sl', 305);  UndoDeleteFcn=plecs('sl', 306);  PreSaveFcn=plecs('sl', 311);  NameChangeFcn=plecs('sl', 310);  DestroyFcn=plecs('sl', 307);  OpenFcn=plecs('sl', 302);  ErrorFcn=plerrorfcn
      mask Display: plot([0.1 0.9 0.9 0.1 0.1], [0.9 0.9 0.5 0.5 0.9])
  Valphabeta : Subsystem  Commented=on  LoadFcn=plecs('sl', 300);  InitFcn=plecs('sl', 314);  StartFcn=plecs('sl', 308);  StopFcn=plecs('sl', 309);  mask{Settings=<binary blob, 236 chars, not shown>}
      mask init:
      | plecs('sl', 315);
      settings: CopyFcn=plecs('sl', 303);  DeleteFcn=plecs('sl', 305);  UndoDeleteFcn=plecs('sl', 306);  PreSaveFcn=plecs('sl', 311);  NameChangeFcn=plecs('sl', 310);  DestroyFcn=plecs('sl', 307);  OpenFcn=plecs('sl', 302);  ErrorFcn=plerrorfcn
      mask Display: plot([0.1 0.9 0.9 0.1 0.1], [0.9 0.9 0.5 0.5 0.9])
  abc to Alpha-Beta-Zero1 : powerlib_meascontrol/Transformations/abc to Alpha-Beta-Zero
  q reference : Step  Time=0  After=0  SampleTime=0
  w0 : Step  Time=0  After=2*pi*50  SampleTime=0
  SRF_freq : Outport
  wires:
  Add1/1 -> Product/2, Integrator/1
  Alpha-Beta-Zero to dq0/1 -> Demux/1
  Constant/1 -> Math Function/2
  Demux/3 -> Terminator/1
  1/(2*pi)/1 -> Product/1
  q reference/1 -> Add/2
  Integrator/1 -> Math Function/1
  Product/1 -> SRF_freq/1
  Add/1 -> Gain/1
  Gain/1 -> PI Controller/1
  w0/1 -> Add1/2
  PI Controller/1 -> Add1/1
  abc to Alpha-Beta-Zero1/1 -> Valphabeta/1(1), Alpha-Beta-Zero to dq0/1
  Math Function/1 -> Alpha-Beta-Zero to dq0/2
  Demux/2 -> Add/1
  Vabc-PLL/1 -> Vabc/1(1), abc to Alpha-Beta-Zero1/1
  Demux/1 -> Terminator1/1

== system ThreePhaseVectorControl/Vector Current Controller + PWM/SRF_PLL/Vabc ==
  1 : Inport
  " InputMux " : Subsystem
      mask Display: disp('Mux')
  " S-Function " : S-Function  FunctionName=plecs  SFunctionDeploymentMode=off  EnableBusSupport=off
  wires:
  1/1 -> " InputMux "/1(In1)
  " InputMux "/1(Out) -> " S-Function "/1

== system ThreePhaseVectorControl/Vector Current Controller + PWM/SRF_PLL/Valphabeta ==
  1 : Inport
  " InputMux " : Subsystem
      mask Display: disp('Mux')
  " S-Function " : S-Function  FunctionName=plecs  SFunctionDeploymentMode=off  EnableBusSupport=off
  wires:
  1/1 -> " InputMux "/1(In1)
  " InputMux "/1(Out) -> " S-Function "/1

== system ThreePhaseVectorControl/Vector Current Controller + PWM/Scope1/ InputMux  ==
  In1 : Inport
  Convert1 : DataTypeConversion  SaturateOnIntegerOverflow=on  RndMeth=Zero
  Mux : Mux  Inputs=1
  Out : Outport
  wires:
  Convert1/1 -> Mux/1
  In1/1 -> Convert1/1
  Mux/1 -> Out/1

== system ThreePhaseVectorControl/Vector Current Controller + PWM/CF/MPM (forcing Vq=0)/SRF_PLL for initialisation ==
  Valpabeta0 : Inport
  Add : Sum  Inputs=+-
  Add1 : Sum
  Alpha-Beta-Zero to dq0 : powerlib_meascontrol/Transformations/Alpha-Beta-Zero to dq0  Alignment=Aligned with phase A axis
  Constant : Constant  Value=2*pi
  Demux : Demux  Outputs=3
  Gain : Gain  Gain=Kp_PLL
  Integrator : Integrator  UpperSaturationLimit=2*pi  LowerSaturationLimit=0  IgnoreLimit=on
  Math Function : Math  Operator=mod  SignedPower=on  SaturateOnIntegerOverflow=on
  PI Controller : TransferFcn  Numerator=[1 Ki_PLL]  Denominator=[1 0]
  Terminator : Terminator
  Terminator1 : Terminator
  q reference : Step  Time=0  After=0  SampleTime=0
  w0 : Step  Time=0  After=2*pi*50  SampleTime=0
  SRF_theta : Outport
  wires:
  Add1/1 -> Integrator/1
  Alpha-Beta-Zero to dq0/1 -> Demux/1
  Constant/1 -> Math Function/2
  Demux/3 -> Terminator/1
  q reference/1 -> Add/2
  Integrator/1 -> Math Function/1
  Add/1 -> Gain/1
  Gain/1 -> PI Controller/1
  w0/1 -> Add1/2
  PI Controller/1 -> Add1/1
  Valpabeta0/1 -> Alpha-Beta-Zero to dq0/1
  Math Function/1 -> SRF_theta/1, Alpha-Beta-Zero to dq0/2
  Demux/2 -> Add/1
  Demux/1 -> Terminator1/1

== system ThreePhaseVectorControl/Vector Current Controller + PWM/CF (2)/Force Vq=0/SRF_PLL for initialisation ==
  Valpabeta0 : Inport
  Add : Sum  Inputs=+-
  Add1 : Sum
  Alpha-Beta-Zero to dq0 : powerlib_meascontrol/Transformations/Alpha-Beta-Zero to dq0  Alignment=Aligned with phase A axis
  Constant : Constant  Value=2*pi
  Demux : Demux  Outputs=3
  Gain : Gain  Gain=Kp_PLL
  Integrator : Integrator  UpperSaturationLimit=2*pi  LowerSaturationLimit=0  IgnoreLimit=on
  Math Function : Math  Operator=mod  SignedPower=on  SaturateOnIntegerOverflow=on
  PI Controller : TransferFcn  Numerator=[1 Ki_PLL]  Denominator=[1 0]
  Terminator : Terminator
  Terminator1 : Terminator
  q reference : Step  Time=0  After=0  SampleTime=0
  w0 : Step  Time=0  After=2*pi*50  SampleTime=0
  SRF_theta : Outport
  wires:
  Add1/1 -> Integrator/1
  Alpha-Beta-Zero to dq0/1 -> Demux/1
  Constant/1 -> Math Function/2
  Demux/3 -> Terminator/1
  q reference/1 -> Add/2
  Integrator/1 -> Math Function/1
  Add/1 -> Gain/1
  Gain/1 -> PI Controller/1
  w0/1 -> Add1/2
  PI Controller/1 -> Add1/1
  Valpabeta0/1 -> Alpha-Beta-Zero to dq0/1
  Math Function/1 -> SRF_theta/1, Alpha-Beta-Zero to dq0/2
  Demux/2 -> Add/1
  Demux/1 -> Terminator1/1

== system ThreePhaseVectorControl/Vector Current Controller + PWM/CF 2/MPM (forcing Vq=0)/SRF-PLL for initialization ==
  VaB0 : Inport
  Add : Sum  Inputs=+-
  Add1 : Sum
  Alpha-Beta-Zero to dq0 : powerlib_meascontrol/Transformations/Alpha-Beta-Zero to dq0  Alignment=Aligned with phase A axis
  Constant : Constant  Value=2*pi
  Demux : Demux  Outputs=3
  Gain : Gain  Gain=Kp_PLL
  Integrator : Integrator  UpperSaturationLimit=2*pi  LowerSaturationLimit=0  IgnoreLimit=on
  Math Function : Math  Operator=mod  SignedPower=on  SaturateOnIntegerOverflow=on
  PI Controller : TransferFcn  Numerator=[1 Ki_PLL]  Denominator=[1 0]
  Terminator : Terminator
  Terminator1 : Terminator
  q reference : Step  Time=0  After=0  SampleTime=0
  w0 : Step  Time=0  After=2*pi*50  SampleTime=0
  SRF_theta : Outport
  wires:
  Demux/2 -> Add/1
  Math Function/1 -> SRF_theta/1, Alpha-Beta-Zero to dq0/2
  PI Controller/1 -> Add1/1
  q reference/1 -> Add/2
  Gain/1 -> PI Controller/1
  w0/1 -> Add1/2
  Demux/3 -> Terminator/1
  Add/1 -> Gain/1
  Alpha-Beta-Zero to dq0/1 -> Demux/1
  Constant/1 -> Math Function/2
  Integrator/1 -> Math Function/1
  Add1/1 -> Integrator/1
  VaB0/1 -> Alpha-Beta-Zero to dq0/1
  Demux/1 -> Terminator1/1

== system ThreePhaseVectorControl/Vector Current Controller + PWM/FFT_PLL/MPM (forcing Vq=0)/SRF-PLL for initialization ==
  VaB0 : Inport
  Add : Sum  Inputs=+-
  Add1 : Sum
  Alpha-Beta-Zero to dq0 : powerlib_meascontrol/Transformations/Alpha-Beta-Zero to dq0  Alignment=Aligned with phase A axis
  Constant : Constant  Value=2*pi
  Demux : Demux  Outputs=3
  Gain : Gain  Gain=Kp_PLL
  Integrator : Integrator  UpperSaturationLimit=2*pi  LowerSaturationLimit=0  IgnoreLimit=on
  Math Function : Math  Operator=mod  SignedPower=on  SaturateOnIntegerOverflow=on
  PI Controller : TransferFcn  Numerator=[1 Ki_PLL]  Denominator=[1 0]
  Terminator : Terminator
  Terminator1 : Terminator
  q reference : Step  Time=0  After=0  SampleTime=0
  w0 : Step  Time=0  After=2*pi*50  SampleTime=0
  SRF_theta : Outport
  wires:
  Demux/2 -> Add/1
  Math Function/1 -> SRF_theta/1, Alpha-Beta-Zero to dq0/2
  PI Controller/1 -> Add1/1
  q reference/1 -> Add/2
  Gain/1 -> PI Controller/1
  w0/1 -> Add1/2
  Demux/3 -> Terminator/1
  Add/1 -> Gain/1
  Alpha-Beta-Zero to dq0/1 -> Demux/1
  Constant/1 -> Math Function/2
  Integrator/1 -> Math Function/1
  Add1/1 -> Integrator/1
  VaB0/1 -> Alpha-Beta-Zero to dq0/1
  Demux/1 -> Terminator1/1

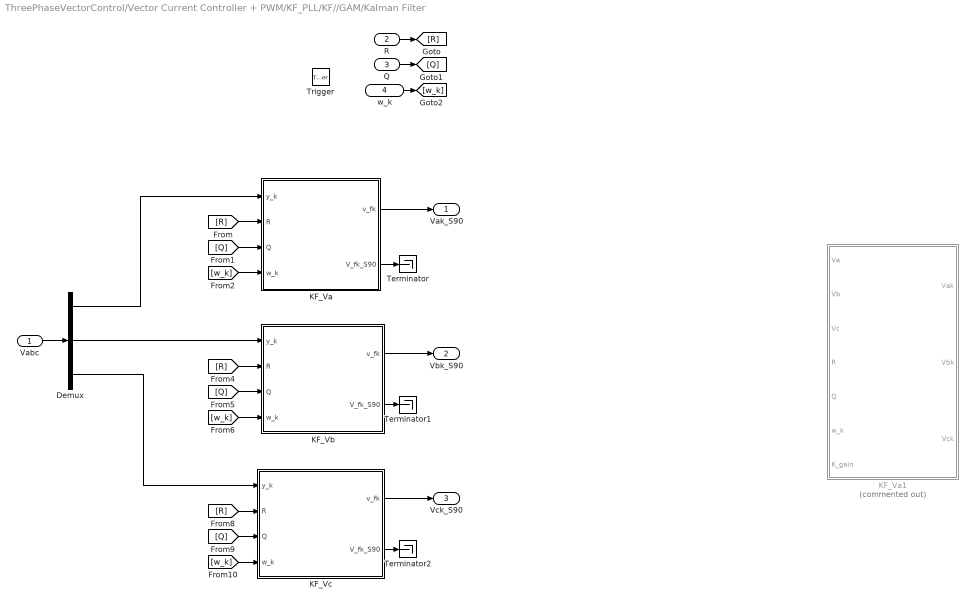
== system ThreePhaseVectorControl/Vector Current Controller + PWM/KF_PLL/KF//GAM/Kalman Filter ==
  Vabc : Inport
  R : Inport  Port=2
  Q : Inport  Port=3
  w_k : Inport  Port=4  LatchByDelayingOutsideSignal=on
  Trigger : TriggerPort  VariantControl=Variant  PortDimensions=1
  Demux : Demux  Outputs=3
  KF_Va : MATLAB Function  TreatAsAtomicUnit=on
  KF_Va1 : MATLAB Function  Commented=on  TreatAsAtomicUnit=on
  KF_Vb : MATLAB Function  TreatAsAtomicUnit=on
  KF_Vc : MATLAB Function  TreatAsAtomicUnit=on
  Terminator : Terminator
  Terminator1 : Terminator
  Terminator2 : Terminator
  Vak_S90 : Outport
  Vbk_S90 : Outport  Port=2
  Vck_S90 : Outport  Port=3
  wires:
  Vabc/1 -> Demux/1
  Demux/1 -> KF_Va/1(y_k)
  R/1 -> [R]
  Q/1 -> [Q]
  w_k/1 -> [w_k]
  [R] -> KF_Va/2(R)
  [Q] -> KF_Va/3(Q)
  [w_k] -> KF_Va/4(w_k)
  [w_k] -> KF_Vb/4(w_k)
  [Q] -> KF_Vb/3(Q)
  [R] -> KF_Vb/2(R)
  [R] -> KF_Vc/2(R)
  [Q] -> KF_Vc/3(Q)
  [w_k] -> KF_Vc/4(w_k)
  Demux/2 -> KF_Vb/1(y_k)
  Demux/3 -> KF_Vc/1(y_k)
  KF_Vc/2(V_fk_S90) -> Terminator2/1
  KF_Vb/2(V_fk_S90) -> Terminator1/1
  KF_Va/2(V_fk_S90) -> Terminator/1
  KF_Va/1(v_fk) -> Vak_S90/1
  KF_Vc/1(v_fk) -> Vck_S90/1
  KF_Vb/1(v_fk) -> Vbk_S90/1

== system ThreePhaseVectorControl/Vector Current Controller + PWM/KF_PLL/KF//GAM/Real Time Frequency Detection ==
  note: $x_{2_k}$
  note: $x_{1_k}$
  note: $\omega_k$
  r1 : Inport
  r2 : Inport  Port=2
  Trigger : TriggerPort  VariantControl=Variant  PortDimensions=1
  Add1 : Sum
  Discrete Derivative : simulink/Discrete/Discrete Derivative  gainval=1.0  ICPrevScaledInput=0  OutMin=[]  OutMax=[]  OutDataType=fixdt(1, 16)  OutScaling=2^-10  DoSatur=off
  Discrete Derivative1 : simulink/Discrete/Discrete Derivative  gainval=1.0  ICPrevScaledInput=0  OutMin=[]  OutMax=[]  OutDataType=fixdt(1, 16)  OutScaling=2^-10  DoSatur=off
  Divide4 : Product  Inputs=/*
  Product3 : Product
  Product4 : Product
  Square2 : Math  Operator=square  SaturateOnIntegerOverflow=on
  Square3 : Math  Operator=square  SaturateOnIntegerOverflow=on
  Subtract1 : Sum  Inputs=+-
  w_k : Outport
  wires:
  Subtract1/1 -> Divide4/2
  Product4/1 -> Subtract1/2
  r2/1 -> Square3/1, Discrete Derivative1/1, Product3/2
  Square3/1 -> Add1/2
  r1/1 -> Discrete Derivative/1, Product4/1, Square2/1
  Product3/1 -> Subtract1/1
  Square2/1 -> Add1/1
  Divide4/1 -> w_k/1
  Add1/1 -> Divide4/1
  Discrete Derivative1/1 -> Product4/2
  Discrete Derivative/1 -> Product3/1

== system ThreePhaseVectorControl/Vector Current Controller + PWM/KF_PLL/KF//GAM/abc-to-aphabetazero and Normalized ==
  note: $||v_{\alpha \beta k}^+||$
  note: $v_{\beta k}^+$
  note: $v_{\alpha k}^+$
  note: $r_{\beta_\omega}=cos(\theta_k^+)$
  note: $r_{\alpha__\omega}=sin(\theta_k^+)$
  note: $||v_{\alpha \beta k}^+||$
  Va S90 : Inport
  Vb S90 : Inport  Port=2
  Vc S90 : Inport  Port=3
  Trigger : TriggerPort  VariantControl=Variant  PortDimensions=1
  Add4 : Sum
  Demux : Demux  Outputs=3
  Divide : Product  Inputs=*/
  Divide2 : Product  Inputs=/*
  Mux : Mux  Inputs=3
  Square Root : Sqrt  SaturateOnIntegerOverflow=on
  Square6 : Math  Operator=square  SaturateOnIntegerOverflow=on
  Square7 : Math  Operator=square  SaturateOnIntegerOverflow=on
  Terminator : Terminator
  abc to Alpha-Beta-Zero : powerlib_meascontrol/Transformations/abc to Alpha-Beta-Zero
  r_bw : Outport
  r_aw : Outport  Port=2
  wires:
  abc to Alpha-Beta-Zero/1 -> Demux/1
  Square Root/1 -> Divide2/1, Divide/2
  Demux/2 -> Divide2/2, Square6/1
  Add4/1 -> Square Root/1
  Square7/1 -> Add4/1
  Square6/1 -> Add4/2
  Demux/1 -> Square7/1, Divide/1
  Demux/3 -> Terminator/1
  Mux/1 -> abc to Alpha-Beta-Zero/1
  Vc S90/1 -> Mux/3
  Divide2/1 -> r_bw/1
  Divide/1 -> r_aw/1
  Va S90/1 -> Mux/1
  Vb S90/1 -> Mux/2

== system ThreePhaseVectorControl/Vector Current Controller + PWM/KF_PLL/Kalman Filter-based PLL/Kalman Filter ==
  Va : Inport
  Vb : Inport  Port=2
  Vc : Inport  Port=3
  R : Inport  Port=4
  Q : Inport  Port=5
  w_fk : Inport  Port=6
  w_k : Inport  Port=7  LatchByDelayingOutsideSignal=on
  Trigger : TriggerPort  VariantControl=Variant  PortDimensions=1
  KF_Va : MATLAB Function  TreatAsAtomicUnit=on
  KF_Vb : MATLAB Function  TreatAsAtomicUnit=on
  KF_Vc : MATLAB Function  TreatAsAtomicUnit=on
  Scope : Scope  NumInputPorts=3
  Scope1 : Scope
  Vak_S90 : Outport
  Vbk_S90 : Outport  Port=2
  Vck_S90 : Outport  Port=3
  wires:
  Va/1 -> KF_Va/1(Va)
  Vb/1 -> KF_Vb/1(Vb)
  Vc/1 -> KF_Vc/1(Vc)
  R/1 -> KF_Vc/2(R), KF_Vb/2(R), KF_Va/2(R)
  Q/1 -> KF_Vc/3(Q), KF_Vb/3(Q), KF_Va/3(Q)
  w_k/1 -> Scope1/1, KF_Vc/4(w_k), KF_Vb/4(w_k), KF_Va/4(w_k)
  w_fk/1 -> KF_Va/5(w_fk), KF_Vb/5(w_fk), KF_Vc/5(w_fk)
  KF_Va/1(Vak_S90) -> Scope/1, Vak_S90/1
  KF_Vb/1(Vbk_S90) -> Scope/2, Vbk_S90/1
  KF_Vc/1(Vck_S90) -> Scope/3, Vck_S90/1
